simulink model "MGDC_Hardware_in_the_Loop"  (R2025b)
settings: Solver=VariableStepAuto  StartTime=0.0  StopTime=50  RelTol=1e-3
undefined symbols (not defined in the file): LF
libraries: instrumentseriallib x3
(part 1 of 3)
settings Model: Creator=joseA  LastModifiedBy=joseA

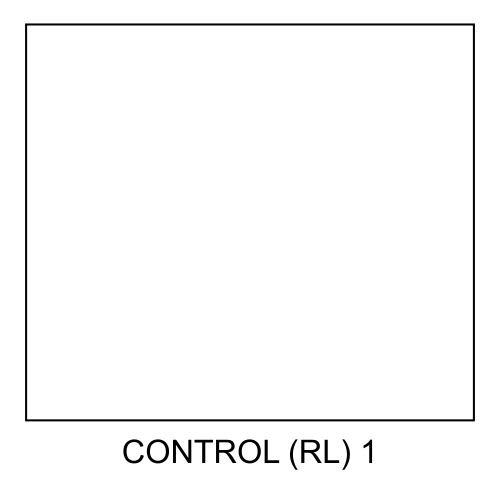
[thumbnail: Simulink's stored preview of the top-level diagram]
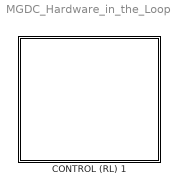
== system MGDC_Hardware_in_the_Loop ==
  CONTROL (RL) 1 : Subsystem

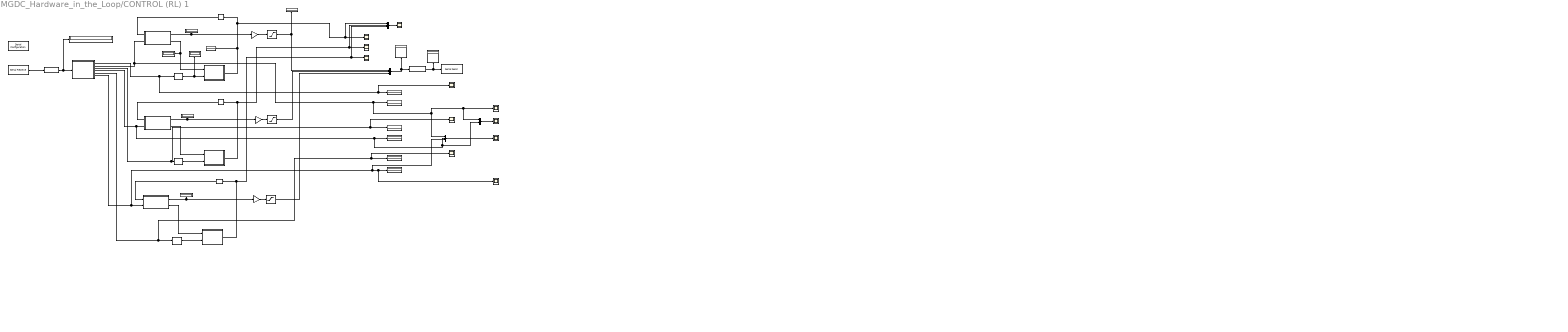
== system MGDC_Hardware_in_the_Loop/CONTROL (RL) 1 ==
  note: Rd1 = 1/100  → convertidor 1 aporta más corriente
      | Rd2 = 1/80
      | Rd3 = 1/60   → convertidor 3 aporta menos corriente
  note: IN_DATA_CONVERTER
  note: Rd1 = 1/100  → convertidor 1 aporta más corriente
      | Rd2 = 1/80
      | Rd3 = 1/60   → convertidor 3 aporta menos corriente
  ASCII to String1 : ASCIIToString
  CORRIENTE convertidor 1 : Display
  CORRIENTE convertidor 2 : Display
  CORRIENTE convertidor 3 : Display
  "Corriente 1 convertidor " : Scope
      settings: ActiveDisplayYMinimum=-0.026624999999999992  ActiveDisplayYMaximum=0.239625  DataLoggingVariableName=ScopeData14
  Corriente 1 convertidores 3 : Scope
      settings: ActiveDisplayYMinimum=-0.042499999999999996  ActiveDisplayYMaximum=0.3825
  Corriente 2 convertidor : Scope
      settings: ActiveDisplayYMinimum=-0.034499999999999989  ActiveDisplayYMaximum=0.2405  DataLoggingVariableName=ScopeData17
  Corriente 3 convertidores : Scope
      settings: ActiveDisplayYMinimum=-0.034624999999999989  ActiveDisplayYMaximum=0.24162499999999998  DataLoggingVariableName=ScopeData6
  Data Type Conversion2 : DataTypeConversion  OutDataTypeStr=uint8  SaturateOnIntegerOverflow=off  RndMeth=Floor
  Delay : Delay  DelayLength=1  InitialCondition=0  UseCircularBuffer=on  SampleTime=0.02
  Delay1 : Delay  DelayLength=1  InitialCondition=0  UseCircularBuffer=on  SampleTime=0.02
  Delay2 : Delay  DelayLength=1  InitialCondition=0  UseCircularBuffer=on  SampleTime=0.02
  Display1 : Display
  Gain : Gain  Gain=21.25
  Gain1 : Gain  Gain=21.25
  Gain2 : Gain  Gain=21.25
  MATLAB Function1 : MATLAB Function  TreatAsAtomicUnit=on
  Mux : Mux  Inputs=3
  Mux1 : Mux  Inputs=3
  Mux4 : Mux  Inputs=2
  Mux5 : Mux  Inputs=3
  Primario Droop : Subsystem
  Primario Droop1 : Subsystem
  Primario Droop2 : Subsystem
  SERIAL RECEIVE1 : instrumentseriallib/Serial Receive  Priority=1  PortSel=COM7  Port=COM7  ComPort=COM7  DataType=uint8  SaveDataType=uint8  ToggleHeader=off  Header=[]  ToggleDataSize=on  DataSize=[1 50]  ToggleTerminator=on  Terminator=Custom terminator  CustomTerminator=[;]  InputFormat=Column major  EnableBlockingMode=on  ActionDataUnavailable=Output last received value  ActionWhenDataUnavailable=Output last received value  CustomValue=0  SampleTime=0.02  SimulateUsing=Interpreted execution  BlockInModel=on  aMode=1  LibraryInUse=instrumentlib
  Saturation : Saturate  UpperLimit=230  LowerLimit=50
  Saturation1 : Saturate  UpperLimit=255  LowerLimit=0
  Saturation2 : Saturate  UpperLimit=255  LowerLimit=0
  Secundario RL : Subsystem
  Secundario RL1 : Subsystem
  Secundario RL2 : Subsystem
  Serial : Display
  Serial Configuration : instrumentseriallib/Serial Configuration  Priority=-200000  PortSel=COM7  Port=COM7  ComPort=COM7  BaudRate=115200  DataBits=8  Parity=none  StopBits=1  ByteOrder=little-endian  FlowControl=none  Timeout=10  SimulateUsing=Interpreted execution  BlockInModel=on  aMode=1
  Serial Send : instrumentseriallib/Serial Send  Priority=1  PortSel=COM7  Port=COM7  ComPort=COM7  Header=[]  Terminator=LF ('\n')  CustomTerminator=[]  EnableBlockingMode=on  SimulateUsing=Interpreted execution  BlockInModel=on  aMode=1
      settings: LibrarySourceBlock=c2000lib/Host Communication/Serial Send
  Serial2 : Display
  Señal de ontrol 3 convertr : Scope
      settings: ActiveDisplayYMinimum=-0.6320586042914641  ActiveDisplayYMaximum=3.6472287338101634
  Señal de ontrol convertidor 1 : Scope
      settings: ActiveDisplayYMinimum=-0.6320586042914641  ActiveDisplayYMaximum=3.6472287338101634  DataLoggingVariableName=ScopeData2
  Señal de ontrol convertidor 2 : Scope
      settings: ActiveDisplayYMinimum=-0.28991250000000035  ActiveDisplayYMaximum=3.6092125000000008  DataLoggingVariableName=ScopeData7
  Señal de ontrol convertidor 3 : Scope
      settings: ActiveDisplayYMinimum=-0.28991250000000035  ActiveDisplayYMaximum=3.6092125000000008  DataLoggingVariableName=ScopeData8
  VOLTAJE convertidor 1 : Display
  VOLTAJE convertidor 2 : Display
  VOLTAJE convertidor 3 : Display
  VOLTAJE convertidor_1 : Scope
      settings: ActiveDisplayYMinimum=-1.3847499999999997  ActiveDisplayYMaximum=12.46275  DataLoggingVariableName=ScopeData3
  VOLTAJE convertidor_2 : Scope
      settings: ActiveDisplayYMinimum=-13.92777536231884  ActiveDisplayYMaximum=13.76722463768116  DataLoggingVariableName=ScopeData4
  VOLTAJE convertidor_3 : Scope
      settings: ActiveDisplayYMinimum=-1.3847499999999997  ActiveDisplayYMaximum=12.46275  DataLoggingVariableName=ScopeData5
  Vo : Display
  Voltaje de control{1..3,6} (4 alike) : Display
  Vs/accion : Display
  Zero-Order Hold1 : ZeroOrderHold  SampleTime=0.01
  Zero-Order Hold2 : ZeroOrderHold  SampleTime=0.01
  Zero-Order Hold3 : ZeroOrderHold  SampleTime=0.01
  ref : Display
  wires:
  Zero-Order Hold1/1 -> Primario Droop/1(vs/accion)
  Secundario RL/1(vs/accion) -> Zero-Order Hold1/1, Mux5/1, Señal de ontrol convertidor 1/1, Vs/accion/1
  Primario Droop/2(ref) -> ref/1, Secundario RL/1(ref)
  Delay/1 -> Secundario RL/2(Vo), Vo/1
  Primario Droop/1(Vp) -> Voltaje de control2/1, Gain/1
  MATLAB Function1/1(V1) -> VOLTAJE convertidor_1/1, VOLTAJE convertidor 1/1, Delay/1
  MATLAB Function1/2(I1) -> CORRIENTE convertidor 1/1, Mux4/1, "Corriente 1 convertidor "/1, Mux1/1, Primario Droop/2(i)
  SERIAL RECEIVE1/1 -> ASCII to String1/1
  ASCII to String1/1 -> Display1/1, MATLAB Function1/1(str)
  Gain/1 -> Saturation/1
  Gain1/1 -> Saturation1/1
  Saturation1/1 -> Mux/2
  MATLAB Function1/4(I2) -> CORRIENTE convertidor 2/1, Mux4/2, Mux1/2, Primario Droop1/2(i)
  MATLAB Function1/3(V2) -> VOLTAJE convertidor_2/1, VOLTAJE convertidor 2/1, Delay1/1
  Primario Droop1/1(Vp) -> Gain1/1, Voltaje de control1/1
  Delay1/1 -> Secundario RL1/2(Vo)
  Primario Droop1/2(ref) -> Secundario RL1/1(ref)
  Secundario RL1/1(vs/accion) -> Mux5/2, Señal de ontrol convertidor 2/1, Zero-Order Hold2/1
  Zero-Order Hold2/1 -> Primario Droop1/1(vs/accion)
  Mux/1 -> Serial2/1, Data Type Conversion2/1
  Data Type Conversion2/1 -> Serial Send/1, Serial/1
  Zero-Order Hold3/1 -> Primario Droop2/1(vs/accion)
  Secundario RL2/1(vs/accion) -> Mux5/3, Señal de ontrol convertidor 3/1, Zero-Order Hold3/1
  Primario Droop2/2(ref) -> Secundario RL2/1(ref)
  Delay2/1 -> Secundario RL2/2(Vo)
  Primario Droop2/1(Vp) -> Voltaje de control3/1, Gain2/1
  Gain2/1 -> Saturation2/1
  MATLAB Function1/6(I3) -> Primario Droop2/2(i), Mux1/3, Corriente 1 convertidores 3/1, CORRIENTE convertidor 3/1
  MATLAB Function1/5(V3) -> VOLTAJE convertidor_3/1, VOLTAJE convertidor 3/1, Delay2/1
  Mux1/1 -> Corriente 3 convertidores/1
  Mux4/1 -> Corriente 2 convertidor/1
  Saturation/1 -> Mux/1, Voltaje de control6/1
  Mux5/1 -> Señal de ontrol 3 convertr/1
  ? -> ?
  Saturation2/1 -> Mux/3

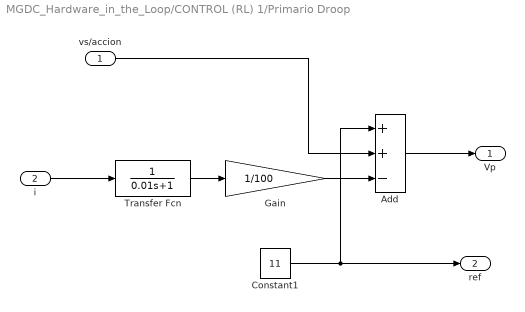
== system MGDC_Hardware_in_the_Loop/CONTROL (RL) 1/Primario Droop ==
  vs/accion : Inport
  i : Inport  Port=2
  Add : Sum  Inputs=++-
  Constant1 : Constant  Value=11
  Gain : Gain  Gain=1/100
  Transfer Fcn : TransferFcn  Denominator=[0.01 1]
  Vp : Outport
  ref : Outport  Port=2
  wires:
  vs/accion/1 -> Add/2
  Transfer Fcn/1 -> Gain/1
  Add/1 -> Vp/1
  Constant1/1 -> Add/1, ref/1
  Gain/1 -> Add/3
  i/1 -> Transfer Fcn/1

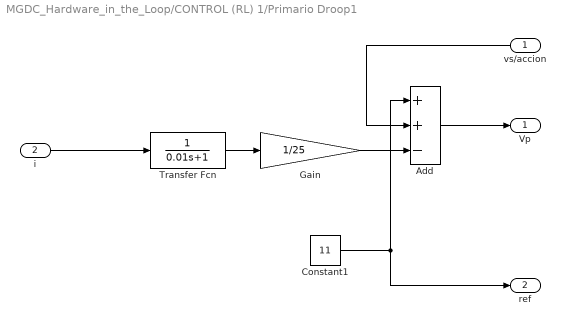
== system MGDC_Hardware_in_the_Loop/CONTROL (RL) 1/Primario Droop1 ==
  vs/accion : Inport
  i : Inport  Port=2
  Add : Sum  Inputs=++-
  Constant1 : Constant  Value=11
  Gain : Gain  Gain=1/25
  Transfer Fcn : TransferFcn  Denominator=[0.01 1]
  Vp : Outport
  ref : Outport  Port=2
  wires:
  i/1 -> Transfer Fcn/1
  Gain/1 -> Add/3
  Constant1/1 -> ref/1, Add/1
  Add/1 -> Vp/1
  Transfer Fcn/1 -> Gain/1
  vs/accion/1 -> Add/2

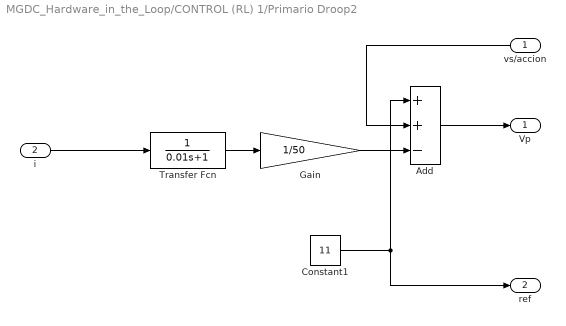
== system MGDC_Hardware_in_the_Loop/CONTROL (RL) 1/Primario Droop2 ==
  vs/accion : Inport
  i : Inport  Port=2
  Add : Sum  Inputs=++-
  Constant1 : Constant  Value=11
  Gain : Gain  Gain=1/50
  Transfer Fcn : TransferFcn  Denominator=[0.01 1]
  Vp : Outport
  ref : Outport  Port=2
  wires:
  vs/accion/1 -> Add/2
  Transfer Fcn/1 -> Gain/1
  Add/1 -> Vp/1
  Constant1/1 -> Add/1, ref/1
  Gain/1 -> Add/3
  i/1 -> Transfer Fcn/1

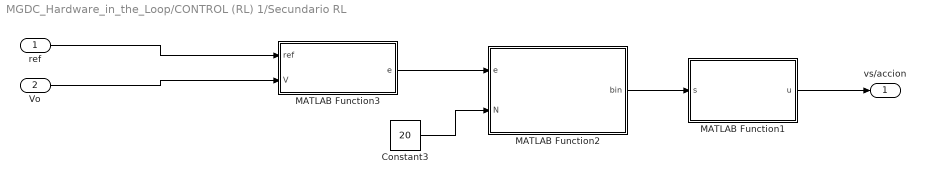
== system MGDC_Hardware_in_the_Loop/CONTROL (RL) 1/Secundario RL ==
  ref : Inport
  Vo : Inport  Port=2
  Constant3 : Constant  Value=20
  MATLAB Function1 : MATLAB Function  TreatAsAtomicUnit=on
  MATLAB Function2 : MATLAB Function  TreatAsAtomicUnit=on
  MATLAB Function3 : MATLAB Function  TreatAsAtomicUnit=on
  vs/accion : Outport
  wires:
  ref/1 -> MATLAB Function3/1(ref)
  Constant3/1 -> MATLAB Function2/2(N)
  MATLAB Function2/1(bin) -> MATLAB Function1/1(s)
  Vo/1 -> MATLAB Function3/2(V)
  MATLAB Function3/1(e) -> MATLAB Function2/1(e)
  MATLAB Function1/1(u) -> vs/accion/1

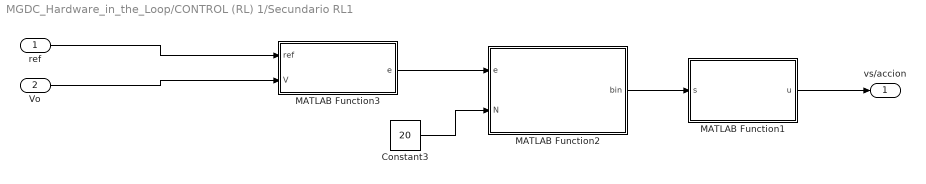
== system MGDC_Hardware_in_the_Loop/CONTROL (RL) 1/Secundario RL1 ==
  ref : Inport
  Vo : Inport  Port=2
  Constant3 : Constant  Value=20
  MATLAB Function1 : MATLAB Function  TreatAsAtomicUnit=on
  MATLAB Function2 : MATLAB Function  TreatAsAtomicUnit=on
  MATLAB Function3 : MATLAB Function  TreatAsAtomicUnit=on
  vs/accion : Outport
  wires:
  MATLAB Function1/1(u) -> vs/accion/1
  MATLAB Function3/1(e) -> MATLAB Function2/1(e)
  Vo/1 -> MATLAB Function3/2(V)
  MATLAB Function2/1(bin) -> MATLAB Function1/1(s)
  Constant3/1 -> MATLAB Function2/2(N)
  ref/1 -> MATLAB Function3/1(ref)

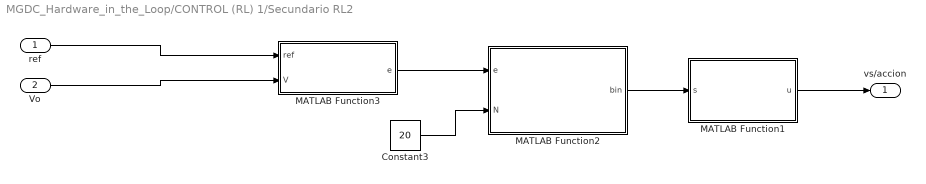
== system MGDC_Hardware_in_the_Loop/CONTROL (RL) 1/Secundario RL2 ==
  ref : Inport
  Vo : Inport  Port=2
  Constant3 : Constant  Value=20
  MATLAB Function1 : MATLAB Function  TreatAsAtomicUnit=on
  MATLAB Function2 : MATLAB Function  TreatAsAtomicUnit=on
  MATLAB Function3 : MATLAB Function  TreatAsAtomicUnit=on
  vs/accion : Outport
  wires:
  ref/1 -> MATLAB Function3/1(ref)
  Constant3/1 -> MATLAB Function2/2(N)
  MATLAB Function2/1(bin) -> MATLAB Function1/1(s)
  Vo/1 -> MATLAB Function3/2(V)
  MATLAB Function3/1(e) -> MATLAB Function2/1(e)
  MATLAB Function1/1(u) -> vs/accion/1

== matlab function MGDC_Hardware_in_the_Loop/CONTROL (RL) 1/Secundario RL/MATLAB Function1 ==
  data: s input; u output
function u = Q_controller(s)

Q = [
-12.7419587257674	-16.5755843510369	-5792.60954433838	-5.76194960479208	-39.0558742239859	-26.3692152815490	-36.7482582683770	-69.2991986569097	-241.468638242565	-119.033145205265	-14.4197256305079	-193.972505342718	-7.49922013095889	-3.43976592786462	-2727.80869189683	-6.57853855354576	-4.67415267221896	-2.86674586110135	-10.8356069237398	-70.7035117726938	-15.2616417811319	-5.89962340573226	-24.2155561499233	-15.8163183273265	-10.5339149563113	-47.6405691387301	-2.07570071479117	-5.37288991207764	-8.98558374248492	-5.85512873224128	-1.84295771751170	-2.83230459467950	-2.29988802171117	-2.61911676537786	-373.245577862944	-2.91193398668742	-5.04616797568849	-2.46245852564098	-1.84790238745244	-1.94907817907462	-1.52029949204548	-812.170681689791	-46.3816310464442	-53.5114564356691	-3.82762960013390	-1.51723982271042	-1.88865621136823	-1.84002611784582	-1.55943343650242	-1.52426557822435	-1.50774921368286	-1.55515768015907	-2.06900168882623	-1.52924123223570	-17.0325035308028	-5.11874537054768	-1.87736420746987	-2.96950386700710	-1.97321137666898	-1.57144844274891	-1084.80181556884	-1.50556483313663	-2.10135942315090	-2.28145516209708	-1.66233446801168	-2.23027478188466	-1.55073923728069	-1.52157258447487	-1.54788431522886	-7.63956360659968	-16.9395672961194	-4.61763699549735	-63.8280439489593	-2.34831771428507	-17.4514437615830	-1.54992585093297	-2.41702833638834	-4.66152255350778	-5202.60935742421	-40.1988565266151	-5.67406404755540	-6.79342614200119	-5.95835907030071	-4.38874189280054	-869.232714982603	-1228.50805533796	-42.0807963277050	-6.01916521114618	-7.48066277911732	-56.0130291493664	-127.066035481111	-5.73898204729753	-2812.14116076311	-2.73744725529453	-198.019171149108	-19.4375133109880	-4.03073055793469	-467.836214097583	-1.68667990256442	-15.1043029284038	-30445.0364631220;
-0.811392102385955	-0.768349080784308	-0.328304456227316	-7.67572202840155	-0.277829845715347	-0.268904020268357	-1.20844253826191	-0.483677059861379	-253.517131117670	-0.418671904830142	-3.01913731859384	-141.985532436589	-2.16947268646069	-1.11151718127110	-0.281765660189905	-0.404827698724585	-65.4563117271309	-0.774053779173750	-0.0836255360689149	-3.40962415617368	-8.79246375336107	-1.81756011147789	-1.06879095898274	-14.4087400257677	-186.849552762060	-1.39654482056967	-0.114064679463399	-0.263935193217876	-0.214007682484725	-0.145728603609883	-0.221051505573673	-0.299727982646811	-7.96333598497380	-0.577113291359272	-0.248879844847067	-0.302203242731317	-0.971680527114807	-0.306588215341276	-0.143325045155836	-0.209956305242517	-0.241023007705104	-0.168428248870619	-0.216999658388015	-0.126919613636737	-0.272562771523336	-0.216949059513267	-0.339267723837838	-0.330666127358898	-0.379838890634021	-0.183686866000955	-0.192792097939807	-0.327117701590555	-0.0829042898136678	-0.0999681440089244	-0.113590126605319	-0.509925724563798	-0.108098354702656	-0.156118713787136	-0.267115080991025	-0.225986651835948	-0.221716004049648	-0.516427637133992	-0.355888029888852	-0.484096775981591	-0.127610769021271	-32791.0690163361	-0.134615664900122	-2.13042117341241	-0.396327022601345	-8.86442043048681	-2.88755886151887	-0.225829818174461	-0.127760583418864	-0.106431758609346	-0.209117770092730	-0.143678215585102	-0.335419628545144	-0.182251201088708	-0.216740735844723	-0.151118030255471	-36.0059634861555	-5.94877505206066	-191.291556779279	-0.388872332495016	-0.412573787308849	-0.729906827539139	-0.641172840257919	-279.011727012501	-31.0868585024589	-2.49043118330487	-0.277938611504953	-0.210929376866326	-0.0956958232369976	-2.07359199161000	-0.186185777553637	-29.7511839666221	-14.3756053791173	-0.223929218071863	-0.192185011598804	-0.505882801104003	-0.503260060080407;
-8.51437725919901	-15.2524998600442	-0.495741160619353	-0.567561072905174	-0.186261457094438	-2.41174020804650	-0.218978042570090	-6.17485503948068	-0.330662281609166	-2.05677855289701	-1.28261995106252	-0.431786467281813	-13.1559294960268	-0.393043266924620	-6.70695649297692	-11.7346500904051	-0.897155946397331	-0.723624841828663	-0.533057953169712	-0.207530991017775	-0.220336697960074	-1.65055701133113	-2.87692160114681	-0.617053223329113	-10.7925965578470	-8.45946582496822	-0.368248138144608	-2.51633130181106	-0.724784328455364	-0.289901001410070	-0.523597293987790	-0.296780963392661	-3.98817206588573	-0.818143821552758	-0.475962004519834	-0.317264489450174	-0.907482471706305	-0.225301868520151	-0.695857969254454	-0.458612222647434	-0.446263048382482	-0.307837974539982	-0.419374263927866	-0.306469324225416	-0.462678385183346	-0.279680347962402	-0.518365448425520	-0.380426431821643	-0.405170924425692	-0.204007351839861	-0.215339422168513	-0.367066349243164	-0.255353091555936	-244.069883525036	-0.235401919867999	-0.351687215877444	-0.269619519146381	-0.423816875564319	-0.202598613561719	-0.519779192987884	-0.182833003171398	-0.376724020996636	-0.438010423037535	-0.207486639709921	-0.639511719044798	-3.52869656787960	-0.626777542139939	-0.355918609453796	-0.576357616345545	-6.15363965426232	-0.287692872514952	-0.467399817064815	-0.792459074886847	-1.84063955498390	-0.232417753059628	-236.769946023068	-2.07827464107265	-0.265696402780039	-3253.95393052357	-0.346916762108799	-0.438826411839273	-1.27626523277912	-0.933945390928540	-0.309037888187083	-15630.9946548075	-0.401533374278553	-6.27521480203173	-0.645405091473676	-2.46658026907137	-49.5916997257110	-0.286795108973196	-0.529150389216740	-0.984125547492295	-0.664897472254698	-1.47605148351359	-0.484952906836338	-1.07428670025658	-898.126809485936	-46.6085267093804	-0.773588637303482	-0.394709963167434;
-0.736059087131580	-0.820374925896869	-1.30404467162199	-1.43475522521622	-1.46617240282116	-0.688493889180265	-0.264575053084401	-0.865704894777033	-0.950953474690836	-0.703724010121451	-1.29163585140073	-1.74662687311797	-0.766655091656393	-2.09280198163952	-1.53924218425000	-0.408529072748902	-0.416152734220584	-247.486279332502	-0.657529786760311	-0.942541651501917	-0.376288231217979	-2.57839616440828	-1.46354444762966	-0.821523121681046	-8.10511891575862	-25.3660815310949	-0.370153542620406	-0.378559021960829	-0.275162703472761	-1.44756864306482	-4.38004599803944	-0.612066553113439	-0.663689140858467	-0.244571648734621	-0.707472382322124	-0.251360037608532	-0.602157206261725	-6.59165015302628	-0.477412174532439	-0.914248931073863	-263.210001491812	-0.527928550292739	-0.321878313042588	-0.471389418246999	-0.414557200120604	-0.275279603664982	-0.386285605169588	-0.327050497049712	-0.361034037987359	-0.349506461953110	-0.527120455223840	-1.24890663554122	-0.359881983205544	-0.358903333494729	-0.405177746872238	-0.330311870605309	-0.502791392504622	-0.379505398130791	-0.370111771988517	-0.480545564238086	-0.226007568127951	-0.899362101319956	-5.03395632028528	-0.297132318809920	-0.514261439939988	-0.338975859301510	-0.353583449021279	-2.39054591309304	-2.02700197824047	-0.919332518816779	-19.2786909001988	-0.672130111077330	-0.551749723885963	-0.550310993349844	-3.54339230169637	-2.44718420181409	-12.2866662405337	-0.486302282745964	-1.45253098698860	-0.238221462304201	-0.224953758412600	-7.42545787293330	-1.73735691817342	-4.40820360800336	-186.929387145588	-0.678695824306881	-0.520361500141342	-0.453245360801098	-11.5629345812393	-19.9818907255171	-0.275497874760507	-6.20641802393820	-53.5980508647647	-0.263293278972767	-0.267818048719752	-0.500771097348248	-6.04481955859599	-2.71319258621081	-1.21079422711117	-0.307358395648242	-5.25738549320229;
-1.20188871419432	-49.6913603535722	-10.9809040825510	-1.98449675345457	-3.16364415623163	-1.98754558410002	-2.79226320762894	-2.05978006855050	-9413.43768644033	-4.48323760400310	-1155.59340752770	-1.87421567546436	-0.575663628971590	-0.625335705722683	-3.58279482927623	-3.88653622654085	-127.936055957864	-0.753522109034835	-12.8483617790880	-9.03412833330472	-2.22559589273954	-2.77453644301501	-1.26046832056643	-0.771011753088913	-12825.2277451568	-0.676420871281627	-0.585367004740776	-1.81033988837519	-7.69144456714536	-97.3961747520477	-4.38722515392629	-6.87188125017945	-1.53963105273380	-0.561917683411952	-0.655843958491068	-2.38243831931505	-0.559493898559097	-2.12230662340186	-1.21266336469103	-256.407123576575	-0.550219563106360	-0.511328849530780	-0.477724973381957	-0.527426217099547	-0.780638919234950	-0.636115320598152	-0.442989819285485	-0.581552284254700	-0.744943382143544	-0.595553632056466	-0.528637815153486	-0.754138312654330	-0.658278128294209	-0.812960726877516	-0.699959535438040	-0.551836192360660	-0.418737136022640	-1.05228394743140	-1.74923676212311	-0.856861247728302	-2.68431182659415	-2.01986926908729	-0.493324177493647	-3.86756682159343	-1.61578282273469	-0.612610410993931	-0.576650868613454	-0.465839714146046	-0.714551849192871	-0.555460129696737	-0.664856663277526	-0.459675554516919	-31.6872770508020	-4.32414065958024	-0.437636570916796	-1.33719930639096	-2.30414651321608	-214.427875210897	-38.5836258904109	-1.68315256544962	-39.3647086825418	-0.851072932103953	-0.632296761741850	-3.32759667289808	-0.700330169454616	-2.52697569400439	-0.916271249582170	-0.915035552332330	-92.1813320937650	-1.78800399867201	-2.44928824067269	-8.67513109207657	-1.10996547364767	-37.8537828167956	-1.30585638626964	-3.51521938877688	-9830.57869857570	-32.3698979666384	-28.2499969913869	-15.8528283610922	-1.73737072505462;
-5.82085348826992	-3.32655945177569	-2.26336565995813	-13.3374898737624	-0.924575983085473	-2.81418646207861	-21.6632202239115	-7.51353379455758	-3779.98239858670	-3.66893249991185	-2.58456959487262	-17.3089538447105	-70.4197762486879	-1.25272329649687	-5.41766015943055	-1.43774910537904	-17.2842964887401	-130.050712164895	-2.36563277507109	-1.30977060363276	-4.91472706693597	-5.79075909854481	-13.2923429337802	-0.944520403527340	-84.2972247208227	-4.59911732274606	-2.46469691731549	-1.15381743751615	-0.879030691854968	-0.834958794614883	-1.36516463147707	-5.31059942280980	-1.13504110600226	-0.851353666265701	-1.50796788793085	-0.884030767296859	-0.871905991294095	-86.0151759284261	-4.18324708027431	-0.968385434473369	-1.01072275632323	-1.30601253391143	-0.912388089542700	-13.6597786959721	-959.362491697954	-0.915541684741328	-2.81654699435002	-1.03335604175561	-0.919995027546424	-19.3220670530828	-0.919626760367598	-1.06788823485194	-1654477.20019008	-0.885320789497404	-1.05360051733681	-0.855726998559931	-0.876786675031217	-1.12191424308034	-2.62797779260389	-1.48604777120665	-1.00356686466844	-0.868879899631780	-6.58558774776734	-1.23238508579406	-1.46015397833572	-191.198148809928	-1.47545692049658	-0.908095375169863	-163.604065683162	-0.999416328107739	-0.994946160696477	-2.91972275448215	-1.01931924500223	-8.24206217814783	-0.993063277426773	-1.19347511417080	-1.75650520196497	-3.28013090960121	-1.40713938130720	-0.907474830395992	-7.63978055454912	-5.62093865716766	-1.25382698291468	-2.52163332800301	-305.481733380150	-2.06840103361770	-1.05129795549518	-0.827560974308034	-0.835075481001984	-3.47491238526228	-29.0491742442695	-2.89754125556290	-3.41062098867143	-19.0012152839925	-46.8465187258719	-4.29387662922700	-1.27677276182006	-14.7830220036595	-10.2518678052999	-1.71711628944024	-6.44759649870019;
-54.5596777865474	-27.4402424649158	-1803.70629116675	-51.8396916591693	-1.38653312676822	-19.7718384114135	-42.0622931690948	-2.46255683840909	-22.6118460500334	-19.6515547885098	-90.4512687474906	-2.88656586081984	-1.63373318400342	-18.3244775398846	-1762.44317871189	-3.21900618642950	-105.997739611643	-3.56722731575476	-60.0920998777600	-46.8528094002160	-7.27292429636099	-144.931319581656	-61.0254474424883	-5.14065854104098	-6.02667923728157	-1.32099288233104	-1.64351187023519	-3.86183430864354	-12.9118453130788	-9.46390422762346	-1.38679895551259	-1.25004853227476	-1.32641735065193	-1.69349947173086	-1.28179793103532	-1.57199338784876	-1.26022366666100	-1.35709957275922	-2.91525733998262	-1.36891797442455	-1.40736926179525	-1.36175699611981	-2.31478039951210	-1.33881989023656	-1.29664683905535	-2.41027686898210	-1.58375733192446	-3.35806855114876	-2.45847909244704	-3.70503708600080	-2.68873859853959	-1.24401918679371	-1.30905492277626	-2.08024076122130	-1.31484511961799	-1.26248885471339	-1.23503312130450	-1.26547033756354	-1.60106487402861	-3.87137974890003	-1.58561065319532	-4.35599151171466	-2.42966016759315	-9.76410055589544	-1.96950182587840	-1.31043537673595	-1.31396483671744	-2.93186670726810	-43.3662930398371	-2.32625456648738	-5.69373462518098	-8.70641703327484	-1.40042041345718	-3.00553908699435	-3.99686168189302	-1.36881476892445	-17.9890993786100	-4.04936845448589	-2.74877460197607	-1.77950656942023	-3.40616391215670	-27.9674505896839	-12.5265108615732	-337.805135601900	-29.2322231732232	-2.37389388777550	-9.14710015840018	-270.593022179078	-5.03677744375671	-1.29951865275527	-234.384903417691	-20351.8398637380	-2.11164917955930	-3.79331917423858	-2.75031813363272	-117.659834106172	-16.6157150254822	-21.1110421083318	-15.2891206730547	-290.294131678192	-5.86108771725225;
-15.8990374385315	-20.3839982699941	-54.7329873029913	-120.392050930730	-50.9718197932918	-740.226804396823	-94.5049980458035	-415.201298716316	-2.68344424492604	-18.9100798408665	-13.6862380654222	-68.3408697287631	-3889.20128776938	-33.5801043623214	-77.1201947014658	-33.9992629644012	-113.189309717212	-4.40959864758690	-1.97558622037659	-5.19984732901443	-63.5155046771652	-37.2581992982070	-19.5399224805152	-3.26148649337874	-29.1646688297278	-395.073178871102	-25.0308734022443	-2.55532463695855	-1.94205375289943	-41610.9845499897	-52.4447791153067	-1.97703960739495	-4.28671057454491	-118.893627173359	-5.68186618833983	-9.63084321344062	-2.50967589502203	-4.00215461739001	-8.61508903767201	-8.25478556489232	-2.42036350299168	-3.33639572865414	-5.48075492152078	-2.17692494274773	-1.92068350280365	-4.90373334958241	-3.81743462162337	-33.3532801326715	-3.38830264158465	-3.76755311897301	-6.06832643383321	-1.74043981662769	-1.76520584738403	-1.75012662698454	-1.74547655795434	-1.74500324284826	-42.5368104792347	-2.21474064803748	-1.77594421904730	-6.83865908125398	-11.9582106006669	-2.58912389394518	-1.97827141416632	-2.62768012787274	-1.74830154639137	-2.00839434755562	-9.67154219319746	-3.90976023318651	-275.241714720054	-37.3123306653590	-2.25019314850981	-10.9107404289839	-399.969938169682	-3.16245124668801	-3.53091066357679	-2.47266056470040	-18.8580802287623	-14.0084751431418	-8.06486760443462	-2.91864774764646	-2.97740058225195	-96.9378636376018	-129.985804594066	-13.6220502625227	-386.268842483397	-32.5172167566591	-11.6562832980368	-2.85041977888526	-22.5223365583250	-8.15736556909627	-16.4327026812548	-40.0938460987625	-1423.14006904998	-17.2629525339159	-19.7239109694875	-242.845650341001	-178.523200458734	-112.442918357843	-27.0260863498207	-4.81683392233473	-56.9285732013354;
-26.7249600225356	-19.3466344692665	-4.32433457536230	-22.6118472154302	-5534.54681359084	-48.6562018000906	-11.7622832444369	-36.8717549133604	-15.3673418827022	-3.00170035155272	-43.9952861407046	-11.3297410626542	-1388.75814522035	-22.1902748694124	-436.328890922733	-12.0936804444166	-982.626218378993	-18.0662761071986	-5.06003442319611	-31.0918382661777	-190.772495797191	-15.3703310561165	-4.14309124424684	-6.23364579346658	-12.3381035727679	-40.3424120521635	-6.76817231147030	-12.6709309190700	-44.0715192964416	-96.2519690674768	-276.508782508049	-16170.3515247359	-2.82480427963126	-5.44114579956681	-163.837195728844	-245.543483110719	-2.12384919409492	-2.83846853312776	-2.60969941162947	-262.489923454380	-30.3367833459680	-3.58978559745731	-2.17759040516948	-7.08316552579980	-2.84562376594808	-17582.5081400397	-8.71468250617177	-2.65421158664689	-2.56127553789765	-18.9810661589305	-2.11423718853858	-1.96237516653877	-12.4368912555336	-13.7977423740432	-2.40667625707849	-1.84827880752380	-2.17910885094556	-2.78375861028897	-6.21968762395297	-7.56595549030397	-10.5155799129644	-31.3276325566707	-65.3802197750273	-4.10206996222414	-7.48886409040808	-93.5868517333301	-2.07412210915401	-2.95221860851113	-5.82700836684252	-184.061019220985	-2.58221723656532	-270075.007395730	-636.229134052987	-11.1777562613107	-5.54001422428043	-12.7158382214201	-8.32822780414614	-380.413088156093	-3.76521931533729	-28.2340024554031	-4.71537627919522	-19.3152534709532	-20579.1507173860	-45.3675430007337	-37.0084521700354	-4.93579293130078	-10.6881194838842	-52.7788600682674	-12.4360247258225	-25.1787495901872	-28.2158098117313	-24.9861364923749	-400.287361155481	-8.85119673110968	-34562.1084836942	-6.43241037643472	-935.428801799817	-60.3907919993487	-989.209443299708	-61.4468010076688	-380.333511731445;
-88.3219597499208	-183.632038637101	-37.8591088310775	-2402.69943849994	-65.4139503623531	-15.2831663191612	-9.17465031270478	-8379.58422216510	-42.8099602700491	-112.517790710750	-11.9311278497853	-522.229443884280	-5.13181189038979	-694.414625980369	-24.1184362044430	-55.5521160185690	-29.4426723147603	-165.719551973181	-24.0555183861069	-30.9931852360613	-20.2619692604924	-4.13116549533891	-54.8035568672169	-58.3811911917231	-32.9912479795541	-494.674337294011	-7791.11153907298	-41.8969316628861	-6.60285231306576	-11.7999622481127	-8.81015758942814	-2.82635014249104	-20.3962873455456	-129.663957850545	-7.72305956251874	-3.37833324462548	-27.8196381445416	-5.93306464487290	-3.74346765303421	-5.84039040352703	-54.5392747068092	-3.28344219242027	-2.83609663814546	-2.47864554067956	-72.1045516207087	-2.23569996190670	-3.46315102167272	-2.22440084502465	-6.58660965445093	-8.91542011429037	-2.72335561194016	-1.89790723953684	-2.43268114806467	-4.87409238220329	-153.012966720010	-174.953731336145	-3.18836956597399	-33.1762257295106	-2.48942407948706	-4.02225024074988	-3.16049451223812	-362.877273536942	-1696.95227029236	-2.39679664502167	-16.6762943968645	-5.80999604381745	-11.2215093110261	-12.5999939338356	-40.8259536706095	-2.30165077859586	-3.33493270289997	-30.0117494999756	-9.04367921282416	-5.13365396596818	-3.37120140416864	-20.7752844547262	-9.79483066760496	-13.3910400471765	-6.45317049727259	-25.6248327298890	-10.3056898654466	-51.2173292872298	-6.59125621742169	-3.46744342385896	-548.986417059752	-10.0498166156929	-37.4526219590952	-31.3358232743571	-8.66606366963762	-81.8308742394524	-19582.6339920858	-996.555088137750	-5.47335485388688	-45.7333066642455	-37.5404646402519	-47.1214891381759	-9.41039708730308	-468.255078299765	-13154.8731748372	-22.0141985092338	-296.950148149440;
-94.5012444519215	-25.4331668931205	-279.871687490543	-15.5899458103860	-20.9507700296820	-27.6364322719649	-2774.59133685928	-8.96436841416157	-7.46099615204187	-55.9279861901986	-256.798902413084	-9.49247970750484	-65.4993972541383	-29.2597001286039	-38.0360166295394	-5.93761391542455	-196.044332269800	-3400.80691958391	-405.555674161988	-2179.79336418187	-18.7023825678433	-14935.7102529330	-169.895630810950	-11.4672092776760	-72.5570662502752	-13.1676756414958	-7.85349495201734	-8.71301207717171	-195.876854919074	-4.04434653363249	-28.7197988269425	-7.44937550951130	-21.0148095523045	-6.51811953581662	-21.1358832159428	-3.63950576171119	-18.9046852841449	-343.557137142141	-3.76396089148786	-7.23557490304556	-6.71793231482660	-5.51736122197177	-5.91935338618203	-4.10971086760589	-72.2460874832264	-2.66630586381449	-4.18642243046604	-10.7391867916140	-3.35862240304261	-3.88551000264815	-1.89317143608522	-4.96369454518639	-278.531983719348	-4.66677500140724	-4.42796057244395	-3.93703642744372	-2.47898983066923	-12.4369024937334	-7.64442170976161	-146.861382305143	-4.49916108443470	-109.462531739188	-13.2915702759159	-8.83914149168947	-3.60788587743618	-7.44089936800056	-4.01150393352202	-133.462432228610	-347619.102753276	-8.67790302273931	-5.71345089229393	-2.91557688124964	-3.38366098231767	-19.5247100866373	-60.3733778917833	-2.97552480443183	-48.9122155783439	-9.17525924259568	-8.77381889229161	-19.8615430225242	-7.12372013068663	-3.11329142064025	-142.459634512010	-659.177451282372	-62.0155467080533	-62.9586715783064	-27.9474763046622	-58.8177852876686	-9.87158147578119	-25.6527264999132	-39.7263045034532	-15.6254817714626	-82.3301886254471	-140.402089767413	-66.5727186739089	-15.9473669814672	-17.2387858293839	-48.6771198922987	-207.786278964314	-56529.9122677030	-326217.535426170;
-29.6865667056685	-32.9020044389956	-9.82592586297494	-77.1175390901634	-500.652136697988	-94746.6101846666	-9.76538913310200	-139.802638747551	-17.6026700557931	-20.3332848258623	-1864.62045264476	-27.7727806580156	-20.8948625292184	-12876.6068502726	-8.05860287966330	-138.880047448846	-51.9499984688941	-29.0770962491386	-2.88261335630111	-5.12994158994882	-11.3722753178667	-3.60091036325514	-13.4187873042583	-3.50954072965463	-76.7030172395504	-7.07546097716613	-165.535723562625	-238.239167767362	-53.1613519966560	-390.617138895025	-4.52881889775741	-4.24112222002841	-3.45740953556993	-6348.69613911594	-527.153719314660	-5.84856956055381	-26044.3470143444	-2.83505308367623	-2.30476014767876	-11.3602829493477	-2.13139210621855	-2.88752856780781	-366.273603369793	-48.1720027927722	-3.01750784754728	-3.37170938425644	-2.11676708449671	-2.17558051062800	-3.17807031181150	-2.27268298834714	-16.6534646348518	-3.25190875944398	-1.91636215826562	-2.17458094682527	-7.82241033416970	-1.87855169670287	-2.62762599640910	-3.58949160895904	-2.79512610070996	-16.2016532982049	-8.35167863460077	-2.05725847192823	-4.29038234954270	-2.26372725506655	-15.6250075106326	-41.9246153545251	-2.36240926025642	-3.50106509692042	-2.21119223503769	-76.9744310785368	-34.7368577388200	-4.15810430263613	-6.87281873093732	-240.233896956794	-2.88178583822043	-7.35346046702535	-37.9883024774054	-151.370164736293	-59.2951206193111	-5.95089912173700	-13.8023691375679	-122.509121405141	-23.5839315697000	-29.2793143784436	-8.05135094473613	-8.13629804264360	-5.37147737217984	-62.1817461198856	-67.7565503258851	-23.0288824569143	-11.6971822380778	-6652.61158327287	-17.5137979441963	-208.738631119551	-7.15766548149563	-14.6371684034878	-46.9342925693021	-5.09091944907572	-16.5607441591931	-10.9671122982202	-189.353470185836;
-8.04214710684108	-6203.41205978171	-7.22691212097575	-389.171681002168	-338.214719494497	-37.0089766185723	-103.598684824617	-29.0310976095332	-9.84996288395639	-6.32053252729206	-203.918185647490	-8.43220828313114	-1474.27938156772	-16.5462191418882	-241.617384575759	-22.7477580844600	-3.04901040427312	-3.61520283885995	-7.62270054405991	-15.3301263920955	-1.90656281747679	-351.458381431448	-96.3262062734509	-2.01766434968509	-1.84224033940862	-3.89541546457183	-12.6879566255908	-2.79929464723171	-2.13683144965557	-112.434189959666	-11.3223808657352	-20.5139302551922	-3.57102228513864	-24.8983854057610	-167.479253327332	-2.22015517795622	-3.05255590023197	-7.49607811864798	-186.638157346756	-1.75422257499942	-5.82630435435288	-1.65175624856006	-1.62597682826985	-1.66316704142021	-1.96689275619928	-1.70199212296505	-102.448526577052	-5.90540989064240	-29.8864087098270	-1.68606555910874	-1.64419651299566	-1.61813169230768	-4.28772731585566	-1.62074990100979	-1.99342313435966	-1.60802857196757	-3.85465334201893	-1.64119356717651	-3.25684492122014	-1276.14576999574	-1.81318656312858	-2.52166369168741	-3.46779507077680	-20.2099464667324	-3.06503097390057	-2.70285786019811	-3.21007886186558	-5.58193329984940	-1.62926526568313	-12.3620391333410	-1.73568164669810	-3.28858729089268	-3.56615270067276	-1.68471477226058	-54.9889355282147	-387.819681194587	-131.547834327662	-16223.2665893790	-3.01193952584474	-28.0757846550539	-5.91421722806353	-11.9922522513355	-4.48172056314258	-6.68075578209477	-9.73477093815688	-16.3455664304074	-39.5272744461672	-9.41958716882460	-55.9044173780885	-2.50980579095384	-4.36406495287068	-7.01384907349287	-8.41821392224911	-382.277116779634	-5.89086513464984	-12.3272066677092	-14.9631040723489	-20.8374488220645	-61.1030127697312	-37.9103402418712	-12.8382341779228;
-10.9513937179363	-28882.3348921903	-20.7928274307312	-10.0602997115319	-107.714411623337	-20.1098397203712	-11.5031100995525	-7949.29755013428	-22.0555733019257	-4.25151408038014	-83.9755738946012	-4.93989061605601	-2.93130099014176	-10.0165923538885	-69414.6493326251	-9.85709099120872	-12.7172634379886	-3.78017778594613	-158.014865694481	-2.17842538728502	-3.39115473720447	-26.0778133195526	-3.03054053145833	-1.98196434804528	-5.17690684733220	-75.1144197642511	-10.2491078087658	-225.043984414620	-5.89634565391302	-1.50273237463329	-6.06043638690166	-3.60910747787251	-1.97650022516744	-3.87728191146193	-6.06827699661170	-1.38758602838995	-3.23770978450871	-5.88809176698250	-119.959221029226	-1.38586187121601	-1.35867441619328	-1.45743299889469	-97.6142872625715	-1.49225719759692	-1.35745882560213	-36.0341056766944	-24.4134034810727	-1.30747025878416	-1.34494054177178	-1.40917025297034	-1.34862079104879	-1.91331543571523	-1.35403049138258	-1.38203499879883	-3.19815925992939	-9.04497591333763	-1.33521024613225	-1.46608609180833	-3.08970867641602	-1.56308636464601	-8.00857163088681	-2.44591549138415	-1.83565226902347	-1.42591931045419	-1.31888210049006	-249.894681845074	-15.3721666705594	-2.38845029138483	-1.36174372803385	-1.90207198568565	-1.87949618232881	-2.47310485145834	-1.41347042825827	-6.83743474118860	-5.78853705208153	-21.4430322797373	-136.020366196890	-2.18309906950387	-325.732718516739	-10.3897750528637	-8.55063303259546	-7.17106695505864	-13.3850061172518	-4.64881023856445	-13.7960483479246	-3.54962586725883	-32.9341449328015	-144.257335070031	-28.3664331800288	-197.103484401251	-7.41289607354306	-2026.01368784572	-150.764936192271	-38.0694985720200	-1.88913472422031	-3.14547904051091	-5.02231432885374	-11.1727753970233	-5.81392370721918	-116.324229824290	-27.4202947285970;
-3.17558509339723	-5.95747953240221	-13.5366731783246	-9.88634847789954	-28.4788789891197	-2.95481969489226	-75119.8190718323	-3.21952447414151	-15.4973512402308	-4.73060076949783	-10.9384937699790	-3.22634175946302	-248.686884277356	-8.50620078175940	-0.814642354470435	-2.55664224978497	-15.1784018586853	-1.57672390396548	-14.8592721126452	-128.209487048994	-0.888625596562763	-6.26172703254669	-3.85089911120372	-27.8032243811275	-22.9144416148654	-349.294386595928	-1.50788009991310	-1.01916067171747	-0.893900758198033	-2.36613835853936	-1.42474500767658	-1716.33842702802	-7.34821893407670	-1.87774482650312	-23.5901742964864	-1.34754519082661	-5.51996525552549	-0.842404162170387	-1.03590885274506	-0.966656998073349	-1.17857546079559	-0.950027630131223	-0.795450232237396	-0.865134470848741	-0.924735052272069	-8.20420872653507	-0.815358926618218	-0.794347436693604	-0.959675090939091	-0.874642979026691	-0.817610046747861	-0.858727080134143	-0.869510758229165	-0.909113356828249	-0.881426374830589	-0.941807985717676	-1.34890529930445	-0.904970825025627	-95.4939492552485	-1.44813554924667	-28.7060525424648	-0.816975137097603	-1.05072534950832	-1.53556776667070	-1.15932739088068	-1.67887701714671	-0.882923830861110	-1.06336832800349	-3.18577213096093	-1.02627271367822	-2.77122327458326	-1.28849313600937	-17.5610446975724	-1.11517543607177	-0.878995174051329	-1.39790236843070	-1.47153215752263	-50.4313884377079	-4.60357367850516	-158.284147811482	-0.903543618656947	-1.35751673274713	-4.35887576379812	-240.594796670536	-2786.25768581465	-2.60927986602263	-13.6784802199144	-544.990191082942	-3.10427130717126	-5.26896189122332	-8.13833675868480	-2.10304651565250	-0.884758244506099	-4.27725039405064	-5.03102195145952	-2.43160486119098	-5.66840248697257	-1081.23596052662	-138.797077750213	-2.52673814136632	-3.83710546985268;
-13.5692716582918	-1.93781020713663	-7.81064237286037	-0.949621187329534	-87.8525143903598	-1.83389002055885	-2.36492454695914	-1.69039777377688	-4.26006651400056	-1.47337387911518	-20.9907448487511	-0.574420117072050	-0.573450894474513	-0.834348326136759	-0.534889945416262	-48.9233159012712	-0.508979252645391	-0.693731217930436	-0.835541021367746	-4.96284405532066	-365141.027687215	-1.73083742168859	-2.18774872172528	-4.61746723558925	-1.34970536498462	-0.875802205672778	-0.507485863247332	-22.0584594369019	-5.43892213851454	-1.67326760303236	-10.2471684091376	-30.6393954326304	-0.531906405627653	-0.539872213383476	-1.57671672687233	-0.787416271417370	-0.597034244566731	-0.681470033327833	-3.08203693404953	-1.36026688838821	-0.559598964753592	-0.826070010372947	-0.522816818396998	-23.6601367553181	-0.539865367337587	-2.39573746171504	-0.695969265715127	-0.632440389567442	-0.753373583002695	-0.631286122932863	-0.639890245462541	-0.673940926866930	-0.795713107857065	-0.501541767166024	-0.502495762462253	-0.597208042208798	-0.833342871392929	-0.874272858014928	-0.610481009655459	-0.665929793921455	-1.15732117305106	-0.560438591797273	-11.3826569879540	-0.588494177450811	-0.687726981403466	-0.634471536072677	-0.758311409555939	-1.57274800710778	-1.52740152823918	-0.511645732264676	-25.0559421177020	-11.4859028201106	-0.655669238168654	-65.2538878439763	-0.590037628526820	-345815.871880786	-2.36903419008576	-0.865011107733854	-2.89369874336312	-22.4379571659595	-502.672829234554	-35.0150981843294	-1.30089452472757	-0.826422765058753	-1.92734533156616	-9.02321226126511	-1.11525492587822	-0.872582053415418	-2.06677241687970	-0.694381449207886	-0.500137762093915	-196.320399784454	-1.30374687978727	-4.45397785699848	-18.6882317649433	-2.50401791742015	-19.8605291776156	-0.708475266003092	-0.876418950938258	-0.499745966125328	-5.94987207453155;
-0.541423575197245	-7.20358483678278	-0.347407017910303	-5.62825927537813	-280.512665343950	-13.8836518135061	-0.955540250219368	-5.41602048011116	-3.88937523461978	-1.14268660609393	-0.679855927991583	-8.28665440601243	-1.40992804310801	-20.9511139588054	-124.424440765597	-5.34918280400300	-1.06041506670382	-0.390337707698940	-2.09098046767135	-1.11556118356239	-1.66573074813452	-0.704669614824028	-2.19347160156643	-0.396299234863654	-0.406812957313420	-1.14682223747186	-0.584072972057171	-0.412314643641403	-1.64712259612494	-2.55475520281930	-3.00961957283759	-0.358596182248029	-0.257824805415017	-2.75998551356301	-0.256882561795686	-0.573669453850931	-6.88876431218939	-0.470244066756049	-0.270825273197656	-0.352661474019218	-0.374311002230743	-2.00680781960796	-3.51836547151789	-7.81933398186007	-0.401473170225175	-0.379828779916276	-0.473113779600146	-0.594766735146940	-0.307169245209303	-0.423928548882963	-0.284433266528536	-0.440102474290596	-0.294654209725970	-0.389083094279850	-0.315005347300529	-0.472462820373158	-0.315438278693552	-0.382173672197264	-0.487803833117443	-0.498491947246496	-0.624018448115717	-3.09419047318337	-0.380527022793608	-0.303025687471240	-25.9434584945870	-0.486355872403191	-2668.54882008231	-0.605651231989989	-1.14661451550055	-16.3278754284219	-0.388100538481142	-0.405421690784048	-0.678868058698788	-1523.64124889454	-1.03829785603699	-0.444728773838898	-11.6339160910059	-0.448272422897992	-0.303478893964927	-0.945199317164725	-19.7878874172422	-18.5720660849549	-0.425323144549923	-0.989253712659820	-0.379549942718315	-0.708208999169801	-0.535548727673559	-12.0910432658027	-0.416074285632895	-2.29489827917588	-4.89321318064658	-0.745419732656412	-0.530516949588843	-0.334246818703256	-0.434545579905257	-119.622784604455	-90.6916324328421	-0.729274746789179	-206.481133657188	-4.55867311576233	-10.8636519053178;
-0.799593248858797	-3789.11840681826	-0.789569087436336	-1.29979641655951	-8.16136513577249	-68.4827534548972	-0.639554736024866	-0.619705691172932	-385.044172400590	-342.101239295393	-0.330910343800034	-0.663109673750014	-4518.69007385636	-0.576009444797686	-0.480242132987025	-0.312817890222320	-17.0664097246463	-0.189879254368658	-0.420256372472854	-0.630089584558024	-0.518521702244629	-0.168651534421610	-0.722398328597088	-0.286751186891872	-1502.99428804268	-0.393351003857048	-0.401195612813718	-3.52009182475819	-0.934645818153774	-0.863775905418165	-1.43911868448518	-0.591777826125821	-0.413989175899631	-0.186033863936362	-0.369364105891695	-0.423377553089063	-0.147505068917168	-0.425149610097682	-0.697752114429157	-0.241473232434846	-0.699269034431719	-0.211267940471040	-0.395778844640849	-0.728545738759885	-0.665171078405401	-0.260539001037802	-0.169728978294170	-0.203958095121248	-0.280498053742688	-0.550715146697711	-0.255826480090846	-0.141818886438890	-0.431305336802230	-0.313102012541466	-0.171254201433039	-0.252449716604213	-0.156911283882056	-0.161257905103407	-0.401086116349713	-0.267924249383022	-0.345218361553994	-0.246712118828463	-0.427399511119343	-1.07558448116424	-0.468363915194627	-0.636700946568017	-1.07626182104667	-0.480963564583283	-252.256610048076	-0.296647258745044	-0.312200446123566	-0.664673327343648	-0.509827812798558	-12.1039028630777	-1.70198008081455	-18.0518987246177	-0.336115697605422	-0.331902337604001	-0.525710873777547	-0.532969683638698	-0.450873112141215	-11.9530293360204	-0.872227959104710	-0.554369608002553	-0.118951970331577	-0.891000257030014	-0.595883097680624	-29.1899941691516	-0.242660507390969	-44.8047995808526	-0.310955772704036	-0.922285072903823	-1.95777099237299	-0.579743192805588	-0.645873536869344	-0.451996940817046	-1.96719941005665	-1.81694132747453	-0.288733092269017	-3.41383885107141	-0.507862650301109;
-0.0982620891178096	-30.4558045754175	-0.304554871188926	-0.622384058549976	-0.964424648221941	-0.520136571235380	-2035.06428824314	-0.884039961721057	-26.7024997334055	-2.43941022801040	-0.320292310416069	-0.265969120294248	-1.31924445927674	-0.479796621909346	-0.433353641276168	-2.44668715663251	-0.204355153132828	-0.680295123023569	-0.121084147331795	-0.228457132583904	-0.148760884573064	-0.149242274262270	-4.27996322068106	-3.36097145111589	-0.378231774464022	-0.654124032057392	-0.660585991052057	-8.36819440655098	-1.08830194344160	-10.0836295138076	-0.0744058146335578	-0.115443190075070	-0.263940790362444	-0.350310321753186	-0.729769501199451	-0.210310402967903	-0.0698141866246283	-0.530922437098349	-0.250328417215249	-12.3966639853012	-0.194464736213770	-2.25199321649461	-0.181355320450108	-0.167880358368533	-0.197244523186521	-0.395893310213197	-0.109516300172880	-0.156952080739462	-0.358803571675749	-0.0784571456358189	-0.361680612229274	-0.182126812392154	-0.108273490428228	-0.203515928705504	-0.177765887007727	-0.475649958065323	-0.270716403063144	-0.0534700602485041	-0.119258968420406	-0.199620439998427	-0.0480845858024224	-0.255712100042414	-0.0576015993086813	-0.167160746159925	-0.656353811975299	-0.214227332740939	-0.389561950637405	-0.172336104801032	-0.153080692905454	-0.275903272656472	-0.350895060166731	-1.80560002342105	-0.222991148501165	-0.875623217471462	-0.208507936403855	-0.138649289570571	-0.339469433807807	-0.239559410259753	-0.301247260350246	-2159.79480294891	-63.2169873612054	-0.423542109478297	-21.1755794798261	-0.196394682622988	-0.669585243392433	-0.209768062584873	-1.18957457935286	-3.75855566061240	-0.103496676431948	-0.0782074332668742	-0.265138626592036	-0.277435181958087	-1.13277177426713	-3.29979005932539	-0.789141042109211	-0.817768402132119	-0.260410081937546	-0.0616431653213905	-2.07350762091922	-0.0919139553722207	-42003.0663414912;
-32.1754590297085	-11.1600034904314	-22.6672053488241	-2.49401526083703	-26.7180804324306	-41.8038929957271	-14.9903629127480	-2972.58692694421	-24.7279749027624	-28.4706907327286	-5.59766230784877	-690.127139929265	-11.8299712988518	-1557.42976432472	-3.76845193718369	-4533.71661668886	-2.28981362917263	-341.593695839163	-6.70434318323770	-3.06679999673706	-16.3200746733186	-1.62533763293328	-91.3888354903403	-2.03477565019706	-2.11663538726133	-44.4498458251809	-43.5267853462121	-175.346526407708	-99.6867636749147	-3.10650197360689	-28.1536822607477	-47.8188695114038	-9.88684524579212	-5.11235516609360	-4.63544251050642	-2.52426943400825	-2.50287850624322	-18.5008308779968	-1.48797707679362	-27.5367867683928	-1.44764521878043	-2.00158477467612	-14.0461917285999	-306.381744222287	-1.40092675561428	-1.43035211553020	-1.53722934299481	-1942.52211861871	-1.43957926321270	-1.45671028111909	-1.41182684926581	-1.40411883830147	-1.43940042139126	-1.40431654273851	-1.51351826893676	-2.08193279164795	-1.43434604151165	-1.44031096581184	-1.44791321472805	-1.43917452246543	-1.95479083570699	-1106.78161277335	-2.83317896367468	-2.54605265443412	-1.45056200396835	-1.39711029241388	-1.39905930140496	-961.901910439315	-7.58750603405929	-2.96897060763729	-2.59397359866022	-1.66077789169105	-4.25324222385219	-4837.45224386284	-5.98391522089220	-7.08845217588303	-2.84225564890697	-37.4481737273522	-24.2148040288917	-3.18972419257410	-42.0652924153728	-2.59014100103463	-3.31685595644833	-17.8130030834044	-2.41140753603279	-4.41704313534772	-453.357447679543	-17.9984781610322	-77.6961491263168	-10.0293107196836	-59.7184530756310	-20.0931397257427	-7.78401406059744	-5.24370660230682	-47.0288254842208	-4.83455239034472	-15.7053694384990	-34.9475312097275	-2.62561683976188	-4.61552708797420	-31.3353790585176
];

actions = -5:0.1:5;

[~, idx] = max(Q(s,:));
a = actions(idx);

persistent u_prev

if isempty(u_prev)
     u_prev = 0;
end

beta = 0.70; % 0.95
u = beta*u_prev + (1-beta)*a;
u_prev = u;
%u=a;
end

== matlab function MGDC_Hardware_in_the_Loop/CONTROL (RL) 1/Secundario RL/MATLAB Function3 ==
  data: ref input; e output; V input
function e = error(ref,V)


e=(ref-V)/ref;

end

== matlab function MGDC_Hardware_in_the_Loop/CONTROL (RL) 1/Secundario RL/MATLAB Function2 ==
  data: e input; bin output; N input
function bin = error_to_bin(e,N)

error_min = -2; % -0.3 o -1 como estaba -0.5
error_max =  2; % 0.3 o 1 como estaba -0.5

error_edges = linspace(error_min, error_max, N+1);


bin = discretize(e, error_edges);

% Protección contra NaN
if isnan(bin)
    if e < error_edges(1)
        bin = 1;
    else
        bin = N;
    end
end
